simulink model "main"  (R2020a)
settings: Solver=FixedStepAuto  StartTime=0.0  StopTime=500  FixedStep=1e-3  RelTol=1e-3
values from neighbouring files (symbols this model uses):
  A = 2.5437    [configuracion.m]
  Cd = 0.31    [configuracion.m]
  d0 = 200    [configuracion.m]
  f = 0.02    [configuracion.m]
  F0 = m*g*sin(theta0)+f*m*g*cos(theta0)+(rho*Cd*A*(v0+w0)^2)/2    [configuracion.m]
  g = 9.81    [configuracion.m]
  K = 1/(rho*Cd*A*(v0+w0))    (= 0.0479562557583)    [configuracion.m]
  K_acc = place(Ac,Bc,p)    [configuracion.m]
  Kp = tau/(tau_bc*K)    (= 100)    [configuracion.m]
  m = 1500    [configuracion.m]
  rho = 1.202    [configuracion.m]
  tau = m/(rho*Cd*A*(v0+w0))    (= 71.9343836374)    [configuracion.m]
  Ti = tau    (= 71.9343836374)    [configuracion.m]
  v0 = 20    [configuracion.m]
libraries: simulink x10
settings Model: PacingRate=0.500000  Creator=FARUMO-SRM  LastModifiedBy=FARUMO-SRM

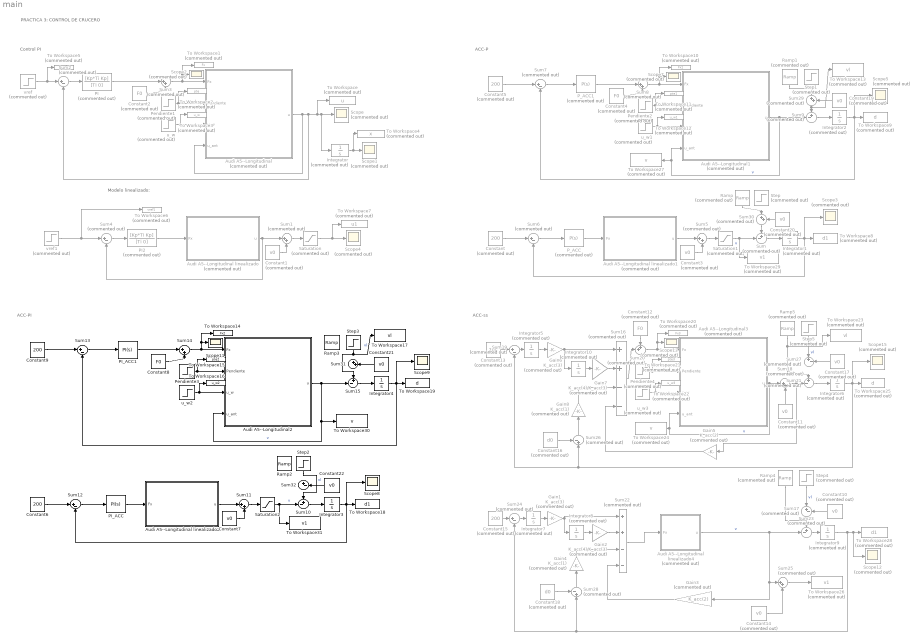
== system main ==
  note: ACC-P
  note: Control PI
  note: PRACTICA 3: CONTROL DE CRUCERO
  note: Modelo linealizado:
  note: ACC-PI
  note: ACC-ss
  Audi A5--Longitudinal : Subsystem  Commented=on
  Audi A5--Longitudinal linealizado : Subsystem  Commented=on
  Audi A5--Longitudinal linealizado1 : Subsystem  Commented=on
  Audi A5--Longitudinal linealizado2 : Subsystem
  Audi A5--Longitudinal linealizado4 : Subsystem  Commented=on
  Audi A5--Longitudinal1 : Subsystem  Commented=on
  Audi A5--Longitudinal2 : Subsystem
  Audi A5--Longitudinal3 : Subsystem  Commented=on
  Constant{,5,13,15} (4 alike) : Constant  Commented=on  Value=200
  Constant{1,3,10..11,14,17,19..20} (8 alike) : Constant  Commented=on  Value=v0
  Constant12 : Constant  Commented=on  Value=F0
  Constant16 : Constant  Commented=on  Value=d0
  Constant18 : Constant  Commented=on  Value=d0
  Constant2 : Constant  Commented=on  Value=F0
  Constant21 : Constant  Value=v0
  Constant22 : Constant  Value=v0
  Constant4 : Constant  Commented=on  Value=F0
  Constant6 : Constant  Value=200
  Constant7 : Constant  Value=v0
  Constant8 : Constant  Value=F0
  Constant9 : Constant  Value=200
  Gain1 : Gain  Commented=on  Gain=K_acc(3)
  Gain2 : Gain  Commented=on  Gain=K_acc(4)/K_acc(3)
  Gain3 : Gain  Commented=on  Gain=K_acc(2)
  Gain4 : Gain  Commented=on  Gain=K_acc(1)
  Gain5 : Gain  Commented=on  Gain=K_acc(2)
  Gain6 : Gain  Commented=on  Gain=K_acc(3)
  Gain7 : Gain  Commented=on  Gain=K_acc(4)/K_acc(3)
  Gain8 : Gain  Commented=on  Gain=K_acc(1)
  Integrator{,5,7..8,10} (5 alike) : Integrator  Commented=on
  Integrator{1..2,6,9} (4 alike) : Integrator  Commented=on  InitialCondition=200
  Integrator3 : Integrator  InitialCondition=200
  Integrator4 : Integrator  InitialCondition=200
  PI : TransferFcn  Commented=on  Numerator=[Kp*Ti Kp]  Denominator=[Ti 0]
  PI2 : TransferFcn  Commented=on  Numerator=[Kp*Ti Kp]  Denominator=[Ti 0]
  PI_ACC : simulink/Continuous/PID Controller  Controller=PI  Form=Parallel  TimeDomain=Continuous-time  UseExternalTs=off  SampleTime=-1  IntegratorMethod=Forward Euler  FilterMethod=Forward Euler  ControllerParametersSource=internal  P=-43.17834467421512  I=-0.01250307588771904  D=0  UseFilter=on  N=100  TunerSelectOption=Transfer Function Based (PID Tuner App)  InitialConditionSource=internal  InitialConditionForIntegrator=0  InitialConditionForFilter=0  DifferentiatorICPrevScaledInput=0  ExternalReset=none  TrackingMode=off  Kt=1  LimitOutput=off  UpperSaturationLimit=inf  LowerSaturationLimit=-inf  LinearizeAsGain=on  AntiWindupMode=none  Kb=1  POutMin=[]  POutMax=[]  IOutMin=[]  IOutMax=[]  DOutMin=[]  DOutMax=[]  NOutMin=[]  NOutMax=[]  SumOutMin=[]  SumOutMax=[]  SaturationOutMin=[]  SaturationOutMax=[]  PParamMin=[]  PParamMax=[]  IParamMin=[]  IParamMax=[]  DParamMin=[]  DParamMax=[]  NParamMin=[]  NParamMax=[]  KbParamMin=[]  KbParamMax=[]  KtParamMin=[]  KtParamMax=[]  KbOutMin=[]  KbOutMax=[]  KtOutMin=[]  KtOutMax=[]  IntegratorOutMin=[]  IntegratorOutMax=[]  FilterOutMin=[]  FilterOutMax=[]  SumI1OutMin=[]  SumI1OutMax=[]  SumI2OutMin=[]  SumI2OutMax=[]  SumI3OutMin=[]  SumI3OutMax=[]  SumI4OutMin=[]  SumI4OutMax=[]  SumDOutMin=[]  SumDOutMax=[]  DifferentiatorOutMin=[]  DifferentiatorOutMax=[]  FilterDiffOutCoefMin=[]  FilterDiffOutCoefMax=[]  ReciprocalOutMin=[]  ReciprocalOutMax=[]  SumDenOutMin=[]  SumDenOutMax=[]  SumNumOutMin=[]  SumNumOutMax=[]  DivideOutMin=[]  DivideOutMax=[]  UdiffTsProdOutMin=[]  UdiffTsProdOutMax=[]  NTsProdOutMin=[]  NTsProdOutMax=[]  UintegralTsProdOutMin=[]  UintegralTsProdOutMax=[]  UngainTsProdOutMin=[]  UngainTsProdOutMax=[]  IntegratorContinuousStateAttributes=''  IntegratorStateMustResolveToSignalObject=off  IntegratorRTWStateStorageClass=Auto  FilterContinuousStateAttributes=''  FilterStateMustResolveToSignalObject=off  FilterRTWStateStorageClass=Auto  ParallelPVariant=InternalParameters  IdealPVariant=Disabled  IVariant=InternalParameters  DVariant=Disabled  IntegratorVariant=Continuous  SatVariant=Disabled  AWVariant=Passthrough  PCopyVariant=Disabled  TRVariant=Disabled  FdbkBlocksVariant=Forward  IdealPFdbkVariant=Disabled  SatFdbkVariant=Disabled  DerivativeFilterVariant=Disabled  NVariant=Disabled  NCopyVariant=Disabled_SignalSpec  FilterICVariant=Disabled  IntegratorICVariant=InternalICs  ExternalResetVariant=Disabled  TRSumVariant=Passthrough  SumFdbkVariant=Disabled  SumVariant=Sum_PI  TsampFilterVariant=InternalTs  TsampNgainVariant=Passthrough  TsampIntegralVariant=Passthrough
  PI_ACC1 : simulink/Continuous/PID Controller  Controller=PI  Form=Parallel  TimeDomain=Continuous-time  UseExternalTs=off  SampleTime=-1  IntegratorMethod=Forward Euler  FilterMethod=Forward Euler  ControllerParametersSource=internal  P=-43.17834467421512  I=-0.01250307588771904  D=0  UseFilter=on  N=100  TunerSelectOption=Transfer Function Based (PID Tuner App)  InitialConditionSource=internal  InitialConditionForIntegrator=0  InitialConditionForFilter=0  DifferentiatorICPrevScaledInput=0  ExternalReset=none  TrackingMode=off  Kt=1  LimitOutput=off  UpperSaturationLimit=inf  LowerSaturationLimit=-inf  LinearizeAsGain=on  AntiWindupMode=none  Kb=1  POutMin=[]  POutMax=[]  IOutMin=[]  IOutMax=[]  DOutMin=[]  DOutMax=[]  NOutMin=[]  NOutMax=[]  SumOutMin=[]  SumOutMax=[]  SaturationOutMin=[]  SaturationOutMax=[]  PParamMin=[]  PParamMax=[]  IParamMin=[]  IParamMax=[]  DParamMin=[]  DParamMax=[]  NParamMin=[]  NParamMax=[]  KbParamMin=[]  KbParamMax=[]  KtParamMin=[]  KtParamMax=[]  KbOutMin=[]  KbOutMax=[]  KtOutMin=[]  KtOutMax=[]  IntegratorOutMin=[]  IntegratorOutMax=[]  FilterOutMin=[]  FilterOutMax=[]  SumI1OutMin=[]  SumI1OutMax=[]  SumI2OutMin=[]  SumI2OutMax=[]  SumI3OutMin=[]  SumI3OutMax=[]  SumI4OutMin=[]  SumI4OutMax=[]  SumDOutMin=[]  SumDOutMax=[]  DifferentiatorOutMin=[]  DifferentiatorOutMax=[]  FilterDiffOutCoefMin=[]  FilterDiffOutCoefMax=[]  ReciprocalOutMin=[]  ReciprocalOutMax=[]  SumDenOutMin=[]  SumDenOutMax=[]  SumNumOutMin=[]  SumNumOutMax=[]  DivideOutMin=[]  DivideOutMax=[]  UdiffTsProdOutMin=[]  UdiffTsProdOutMax=[]  NTsProdOutMin=[]  NTsProdOutMax=[]  UintegralTsProdOutMin=[]  UintegralTsProdOutMax=[]  UngainTsProdOutMin=[]  UngainTsProdOutMax=[]  IntegratorContinuousStateAttributes=''  IntegratorStateMustResolveToSignalObject=off  IntegratorRTWStateStorageClass=Auto  FilterContinuousStateAttributes=''  FilterStateMustResolveToSignalObject=off  FilterRTWStateStorageClass=Auto  ParallelPVariant=InternalParameters  IdealPVariant=Disabled  IVariant=InternalParameters  DVariant=Disabled  IntegratorVariant=Continuous  SatVariant=Disabled  AWVariant=Passthrough  PCopyVariant=Disabled  TRVariant=Disabled  FdbkBlocksVariant=Forward  IdealPFdbkVariant=Disabled  SatFdbkVariant=Disabled  DerivativeFilterVariant=Disabled  NVariant=Disabled  NCopyVariant=Disabled_SignalSpec  FilterICVariant=Disabled  IntegratorICVariant=InternalICs  ExternalResetVariant=Disabled  TRSumVariant=Passthrough  SumFdbkVariant=Disabled  SumVariant=Sum_PI  TsampFilterVariant=InternalTs  TsampNgainVariant=Passthrough  TsampIntegralVariant=Passthrough
  P_ACC : simulink/Continuous/PID Controller  Commented=on  Controller=P  Form=Parallel  TimeDomain=Continuous-time  UseExternalTs=off  SampleTime=-1  IntegratorMethod=Forward Euler  FilterMethod=Forward Euler  ControllerParametersSource=internal  P=-8.95543777959224  I=1  D=0  UseFilter=on  N=100  TunerSelectOption=Transfer Function Based (PID Tuner App)  InitialConditionSource=internal  InitialConditionForIntegrator=0  InitialConditionForFilter=0  DifferentiatorICPrevScaledInput=0  ExternalReset=none  TrackingMode=off  Kt=1  LimitOutput=off  UpperSaturationLimit=inf  LowerSaturationLimit=-inf  LinearizeAsGain=on  AntiWindupMode=none  Kb=1  POutMin=[]  POutMax=[]  IOutMin=[]  IOutMax=[]  DOutMin=[]  DOutMax=[]  NOutMin=[]  NOutMax=[]  SumOutMin=[]  SumOutMax=[]  SaturationOutMin=[]  SaturationOutMax=[]  PParamMin=[]  PParamMax=[]  IParamMin=[]  IParamMax=[]  DParamMin=[]  DParamMax=[]  NParamMin=[]  NParamMax=[]  KbParamMin=[]  KbParamMax=[]  KtParamMin=[]  KtParamMax=[]  KbOutMin=[]  KbOutMax=[]  KtOutMin=[]  KtOutMax=[]  IntegratorOutMin=[]  IntegratorOutMax=[]  FilterOutMin=[]  FilterOutMax=[]  SumI1OutMin=[]  SumI1OutMax=[]  SumI2OutMin=[]  SumI2OutMax=[]  SumI3OutMin=[]  SumI3OutMax=[]  SumI4OutMin=[]  SumI4OutMax=[]  SumDOutMin=[]  SumDOutMax=[]  DifferentiatorOutMin=[]  DifferentiatorOutMax=[]  FilterDiffOutCoefMin=[]  FilterDiffOutCoefMax=[]  ReciprocalOutMin=[]  ReciprocalOutMax=[]  SumDenOutMin=[]  SumDenOutMax=[]  SumNumOutMin=[]  SumNumOutMax=[]  DivideOutMin=[]  DivideOutMax=[]  UdiffTsProdOutMin=[]  UdiffTsProdOutMax=[]  NTsProdOutMin=[]  NTsProdOutMax=[]  UintegralTsProdOutMin=[]  UintegralTsProdOutMax=[]  UngainTsProdOutMin=[]  UngainTsProdOutMax=[]  IntegratorContinuousStateAttributes=''  IntegratorStateMustResolveToSignalObject=off  IntegratorRTWStateStorageClass=Auto  FilterContinuousStateAttributes=''  FilterStateMustResolveToSignalObject=off  FilterRTWStateStorageClass=Auto  ParallelPVariant=InternalParameters  IdealPVariant=Disabled  IVariant=Disabled  DVariant=Disabled  IntegratorVariant=Disabled  SatVariant=Disabled  AWVariant=Disabled  PCopyVariant=Disabled  TRVariant=Disabled  FdbkBlocksVariant=Forward  IdealPFdbkVariant=Disabled  SatFdbkVariant=Disabled  DerivativeFilterVariant=Disabled  NVariant=Disabled  NCopyVariant=Disabled_SignalSpec  FilterICVariant=Disabled  IntegratorICVariant=Disabled  ExternalResetVariant=Disabled  TRSumVariant=Passthrough  SumFdbkVariant=Disabled  SumVariant=Passthrough_P  TsampFilterVariant=InternalTs  TsampNgainVariant=Passthrough  TsampIntegralVariant=Disabled_SignalSpec
  P_ACC1 : simulink/Continuous/PID Controller  Commented=on  Controller=P  Form=Parallel  TimeDomain=Continuous-time  UseExternalTs=off  SampleTime=-1  IntegratorMethod=Forward Euler  FilterMethod=Forward Euler  ControllerParametersSource=internal  P=-8.95543777959224  I=1  D=0  UseFilter=on  N=100  TunerSelectOption=Transfer Function Based (PID Tuner App)  InitialConditionSource=internal  InitialConditionForIntegrator=0  InitialConditionForFilter=0  DifferentiatorICPrevScaledInput=0  ExternalReset=none  TrackingMode=off  Kt=1  LimitOutput=off  UpperSaturationLimit=inf  LowerSaturationLimit=-inf  LinearizeAsGain=on  AntiWindupMode=none  Kb=1  POutMin=[]  POutMax=[]  IOutMin=[]  IOutMax=[]  DOutMin=[]  DOutMax=[]  NOutMin=[]  NOutMax=[]  SumOutMin=[]  SumOutMax=[]  SaturationOutMin=[]  SaturationOutMax=[]  PParamMin=[]  PParamMax=[]  IParamMin=[]  IParamMax=[]  DParamMin=[]  DParamMax=[]  NParamMin=[]  NParamMax=[]  KbParamMin=[]  KbParamMax=[]  KtParamMin=[]  KtParamMax=[]  KbOutMin=[]  KbOutMax=[]  KtOutMin=[]  KtOutMax=[]  IntegratorOutMin=[]  IntegratorOutMax=[]  FilterOutMin=[]  FilterOutMax=[]  SumI1OutMin=[]  SumI1OutMax=[]  SumI2OutMin=[]  SumI2OutMax=[]  SumI3OutMin=[]  SumI3OutMax=[]  SumI4OutMin=[]  SumI4OutMax=[]  SumDOutMin=[]  SumDOutMax=[]  DifferentiatorOutMin=[]  DifferentiatorOutMax=[]  FilterDiffOutCoefMin=[]  FilterDiffOutCoefMax=[]  ReciprocalOutMin=[]  ReciprocalOutMax=[]  SumDenOutMin=[]  SumDenOutMax=[]  SumNumOutMin=[]  SumNumOutMax=[]  DivideOutMin=[]  DivideOutMax=[]  UdiffTsProdOutMin=[]  UdiffTsProdOutMax=[]  NTsProdOutMin=[]  NTsProdOutMax=[]  UintegralTsProdOutMin=[]  UintegralTsProdOutMax=[]  UngainTsProdOutMin=[]  UngainTsProdOutMax=[]  IntegratorContinuousStateAttributes=''  IntegratorStateMustResolveToSignalObject=off  IntegratorRTWStateStorageClass=Auto  FilterContinuousStateAttributes=''  FilterStateMustResolveToSignalObject=off  FilterRTWStateStorageClass=Auto  ParallelPVariant=InternalParameters  IdealPVariant=Disabled  IVariant=Disabled  DVariant=Disabled  IntegratorVariant=Disabled  SatVariant=Disabled  AWVariant=Disabled  PCopyVariant=Disabled  TRVariant=Disabled  FdbkBlocksVariant=Forward  IdealPFdbkVariant=Disabled  SatFdbkVariant=Disabled  DerivativeFilterVariant=Disabled  NVariant=Disabled  NCopyVariant=Disabled_SignalSpec  FilterICVariant=Disabled  IntegratorICVariant=Disabled  ExternalResetVariant=Disabled  TRSumVariant=Passthrough  SumFdbkVariant=Disabled  SumVariant=Passthrough_P  TsampFilterVariant=InternalTs  TsampNgainVariant=Passthrough  TsampIntegralVariant=Disabled_SignalSpec
  Pendiente1 : Step  Commented=on  Time=50  After=0  SampleTime=0
  Pendiente2 : Step  Commented=on  Time=50  After=0  SampleTime=0
  Pendiente3 : Step  Time=50  After=0  SampleTime=0
  Pendiente4 : Step  Commented=on  Time=50  After=0  SampleTime=0
  Ramp{,1,4..5} (4 alike) : simulink/Sources/Ramp  Commented=on  slope=1  start=100  InitialOutput=0
  Ramp2 : simulink/Sources/Ramp  slope=1  start=100  InitialOutput=0
  Ramp3 : simulink/Sources/Ramp  slope=1  start=100  InitialOutput=0
  Saturation : Saturate  Commented=on  UpperLimit=inf  LowerLimit=0
  Saturation1 : Saturate  Commented=on  UpperLimit=inf  LowerLimit=0
  Saturation2 : Saturate  UpperLimit=inf  LowerLimit=0
  Scope{,1..5,7,12..13,15} (10 alike) : Scope  Commented=on
  Scope11 : Scope
  Scope8 : Scope
  Scope9 : Scope
  Step{,1,4..5} (4 alike) : Step  Commented=on  Time=100  Before=20  After=22  SampleTime=0
  Step2 : Step  Time=100  Before=20  After=22  SampleTime=0
  Step3 : Step  Time=100  Before=20  After=22  SampleTime=0
  Sum{,9,21,23} (4 alike) : Sum  Commented=on  Inputs=+-|
  Sum{1,3,5,8,25,29..30} (7 alike) : Sum  Commented=on  Inputs=|++
  Sum10 : Sum  Inputs=+-|
  Sum11 : Sum  Inputs=|++
  Sum12 : Sum  Inputs=|+-
  Sum13 : Sum  Inputs=|+-
  Sum14 : Sum  Inputs=|++
  Sum15 : Sum  Inputs=+-|
  Sum16 : Sum  Commented=on  Inputs=++--
  Sum{2,4,6..7,17..19,24,27} (9 alike) : Sum  Commented=on  Inputs=|+-
  Sum20 : Sum  Commented=on  Inputs=++|
  Sum22 : Sum  Commented=on  Inputs=++--
  Sum26 : Sum  Commented=on  Inputs=-+|
  Sum28 : Sum  Commented=on  Inputs=-+|
  Sum31 : Sum  Inputs=|++
  Sum32 : Sum  Inputs=|+-
  To Workspace : ToWorkspace  Commented=on  VariableName=u  SaveFormat=Timeseries  SampleTime=-1
  To Workspace1 : ToWorkspace  Commented=on  VariableName=Fx  SaveFormat=Timeseries  SampleTime=-1
  To Workspace10 : ToWorkspace  Commented=on  VariableName=Fx1  SaveFormat=Timeseries  SampleTime=-1
  To Workspace11 : ToWorkspace  Commented=on  VariableName=pte1  SaveFormat=Timeseries  SampleTime=-1
  To Workspace12 : ToWorkspace  Commented=on  VariableName=u_w1  SaveFormat=Timeseries  SampleTime=-1
  To Workspace13 : ToWorkspace  Commented=on  VariableName=vl  SaveFormat=Timeseries  SampleTime=-1
  To Workspace14 : ToWorkspace  VariableName=Fx2  SaveFormat=Timeseries  SampleTime=-1
  To Workspace15 : ToWorkspace  VariableName=pte2  SaveFormat=Timeseries  SampleTime=-1
  To Workspace16 : ToWorkspace  VariableName=u_w2  SaveFormat=Timeseries  SampleTime=-1
  To Workspace17 : ToWorkspace  VariableName=vl  SaveFormat=Timeseries  SampleTime=-1
  To Workspace18 : ToWorkspace  VariableName=d1  SaveFormat=Timeseries  SampleTime=-1
  To Workspace19 : ToWorkspace  VariableName=d  SaveFormat=Timeseries  SampleTime=-1
  To Workspace2 : ToWorkspace  Commented=on  VariableName=pte  SaveFormat=Timeseries  SampleTime=-1
  To Workspace20 : ToWorkspace  Commented=on  VariableName=Fx3  SaveFormat=Timeseries  SampleTime=-1
  To Workspace21 : ToWorkspace  Commented=on  VariableName=pte3  SaveFormat=Timeseries  SampleTime=-1
  To Workspace22 : ToWorkspace  Commented=on  VariableName=u_w3  SaveFormat=Timeseries  SampleTime=-1
  To Workspace23 : ToWorkspace  Commented=on  VariableName=vl  SaveFormat=Timeseries  SampleTime=-1
  To Workspace24 : ToWorkspace  Commented=on  VariableName=v  SaveFormat=Timeseries  SampleTime=-1
  To Workspace25 : ToWorkspace  Commented=on  VariableName=d  SaveFormat=Timeseries  SampleTime=-1
  To Workspace26 : ToWorkspace  Commented=on  VariableName=v1  SaveFormat=Timeseries  SampleTime=-1
  To Workspace27 : ToWorkspace  Commented=on  VariableName=v  SaveFormat=Timeseries  SampleTime=-1
  To Workspace28 : ToWorkspace  Commented=on  VariableName=d1  SaveFormat=Timeseries  SampleTime=-1
  To Workspace29 : ToWorkspace  Commented=on  VariableName=v1  SaveFormat=Timeseries  SampleTime=-1
  To Workspace3 : ToWorkspace  Commented=on  VariableName=u_w  SaveFormat=Timeseries  SampleTime=-1
  To Workspace30 : ToWorkspace  VariableName=v  SaveFormat=Timeseries  SampleTime=-1
  To Workspace31 : ToWorkspace  VariableName=v1  SaveFormat=Timeseries  SampleTime=-1
  To Workspace4 : ToWorkspace  Commented=on  VariableName=x  SaveFormat=Timeseries  SampleTime=-1
  To Workspace5 : ToWorkspace  Commented=on  VariableName=vref  SaveFormat=Timeseries  SampleTime=-1
  To Workspace6 : ToWorkspace  Commented=on  VariableName=vref1  SaveFormat=Timeseries  SampleTime=-1
  To Workspace7 : ToWorkspace  Commented=on  VariableName=u1  SaveFormat=Timeseries  SampleTime=-1
  To Workspace8 : ToWorkspace  Commented=on  VariableName=d1  SaveFormat=Timeseries  SampleTime=-1
  To Workspace9 : ToWorkspace  Commented=on  VariableName=d  SaveFormat=Timeseries  SampleTime=-1
  u_w : Step  Commented=on  Time=50  Before=2  After=2  SampleTime=0
  u_w1 : Step  Commented=on  Time=50  Before=2  After=2  SampleTime=0
  u_w2 : Step  Time=50  Before=2  After=2  SampleTime=0
  u_w3 : Step  Commented=on  Time=50  Before=2  After=2  SampleTime=0
  vref : Step  Commented=on  Time=50  Before=20  After=30  SampleTime=0
  vref1 : Step  Commented=on  Time=50  After=10  SampleTime=0
  wires:
  u_w/1 -> Audi A5--Longitudinal/3(u_w), To Workspace3/1
  Pendiente1/1 -> To Workspace2/1, Audi A5--Longitudinal/2(Pendiente)
  Integrator/1 -> To Workspace4/1, Scope1/1
  Sum2/1 -> PI/1
  Sum1/1 -> Saturation/1
  Constant1/1 -> Sum1/2
  Saturation/1 -> To Workspace7/1, Scope4/1
  vref/1 -> To Workspace5/1, Sum2/1
  Audi A5--Longitudinal/1(u) -> Sum2/2, To Workspace/1, Integrator/1, Scope/1, Audi A5--Longitudinal/4(u_ant)
  PI/1 -> Sum3/1
  Sum3/1 -> To Workspace1/1, Scope2/1, Audi A5--Longitudinal/1(Fx)
  Constant2/1 -> Sum3/2
  Audi A5--Longitudinal linealizado/1(u) -> Sum1/1, Sum4/2
  vref1/1 -> Sum4/1, To Workspace6/1
  Sum4/1 -> PI2/1
  PI2/1 -> Audi A5--Longitudinal linealizado/1(Fx)
  Constant3/1 -> Sum5/2
  Sum5/1 -> Saturation1/1
  Saturation1/1 -> To Workspace29/1, Sum/2  "v"
  Audi A5--Longitudinal linealizado1/1(u) -> Sum5/1
  Sum/1 -> Integrator1/1
  Integrator1/1 -> Scope3/1, Sum6/2, To Workspace8/1
  P_ACC/1 -> Audi A5--Longitudinal linealizado1/1(Fx)
  Sum6/1 -> P_ACC/1
  Constant/1 -> Sum6/1
  Sum8/1 -> To Workspace10/1, Scope7/1, Audi A5--Longitudinal1/1(Fx)
  Constant4/1 -> Sum8/2
  P_ACC1/1 -> Sum8/1
  Constant5/1 -> Sum7/1
  Sum7/1 -> P_ACC1/1
  Pendiente2/1 -> To Workspace11/1, Audi A5--Longitudinal1/2(Pendiente)
  u_w1/1 -> Audi A5--Longitudinal1/3(u_w), To Workspace12/1
  Integrator2/1 -> Sum7/2, Scope5/1, To Workspace9/1
  Audi A5--Longitudinal1/1(u) -> Sum9/2, To Workspace27/1, Audi A5--Longitudinal1/4(u_ant)  "v"
  Sum9/1 -> Integrator2/1
  Sum12/1 -> PI_ACC/1
  Sum13/1 -> PI_ACC1/1
  Sum15/1 -> Integrator4/1
  Sum10/1 -> Integrator3/1
  Audi A5--Longitudinal2/1(u) -> Sum15/2, To Workspace30/1, Audi A5--Longitudinal2/4(u_ant)  "v"
  Audi A5--Longitudinal linealizado2/1(u) -> Sum11/1
  Constant9/1 -> Sum13/1
  u_w2/1 -> Audi A5--Longitudinal2/3(u_w), To Workspace16/1
  PI_ACC/1 -> Audi A5--Longitudinal linealizado2/1(Fx)
  Pendiente3/1 -> To Workspace15/1, Audi A5--Longitudinal2/2(Pendiente)
  Integrator4/1 -> Sum13/2, Scope9/1, To Workspace19/1
  Constant8/1 -> Sum14/2
  Sum14/1 -> To Workspace14/1, Scope11/1, Audi A5--Longitudinal2/1(Fx)
  Integrator3/1 -> Scope8/1, Sum12/2, To Workspace18/1
  Constant6/1 -> Sum12/1
  Sum11/1 -> Saturation2/1
  PI_ACC1/1 -> Sum14/1
  Constant7/1 -> Sum11/2
  Saturation2/1 -> To Workspace31/1, Sum10/2  "v"
  Audi A5--Longitudinal3/1(u) -> Sum18/1, Audi A5--Longitudinal3/4(u_ant), To Workspace24/1  "v"
  Sum20/1 -> To Workspace20/1, Scope13/1, Audi A5--Longitudinal3/1(Fx)
  Pendiente4/1 -> To Workspace21/1, Audi A5--Longitudinal3/2(Pendiente)
  Constant13/1 -> Sum19/1
  u_w3/1 -> Audi A5--Longitudinal3/3(u_w), To Workspace22/1
  Sum21/1 -> Integrator6/1
  Sum19/1 -> Integrator5/1
  Sum24/1 -> Integrator7/1
  Integrator9/1 -> Sum28/2, Sum24/2, Scope12/1, To Workspace28/1
  Integrator7/1 -> Gain1/1
  Constant15/1 -> Sum24/1
  Gain3/1 -> Sum22/4
  Sum23/1 -> Integrator9/1
  Gain4/1 -> Sum22/3
  Sum22/1 -> Audi A5--Longitudinal linealizado4/1(Fx)
  Integrator8/1 -> Gain2/1
  Audi A5--Longitudinal linealizado4/1(u) -> Sum25/1, Gain3/1, Sum23/2  "v"
  Integrator6/1 -> Sum26/2, Sum19/2, Scope15/1, To Workspace25/1
  Gain7/1 -> Sum16/2
  Integrator5/1 -> Gain6/1
  Integrator10/1 -> Gain7/1
  Gain5/1 -> Sum16/4
  Gain8/1 -> Sum16/3
  Gain1/1 -> Sum22/1, Integrator8/1
  Gain6/1 -> Sum16/1, Integrator10/1
  Sum16/1 -> Sum20/2
  Gain2/1 -> Sum22/2
  Sum18/1 -> Gain5/1, Sum21/2
  Constant11/1 -> Sum18/2
  Sum26/1 -> Gain8/1
  Constant12/1 -> Sum20/1
  Constant16/1 -> Sum26/1
  Constant17/1 -> Sum27/2
  Constant18/1 -> Sum28/1
  Sum28/1 -> Gain4/1
  Constant10/1 -> Sum17/2
  Step4/1 -> Sum17/1  "vl"
  Constant14/1 -> Sum25/2
  Sum25/1 -> To Workspace26/1
  Step5/1 -> Sum27/1  "vl"
  Constant19/1 -> Sum29/2
  Ramp5/1 -> Sum21/1, To Workspace23/1
  Ramp4/1 -> Sum23/1
  Ramp1/1 -> Sum29/1
  Sum29/1 -> To Workspace13/1, Sum9/1
  Ramp/1 -> Sum30/1
  Sum30/1 -> Sum/1
  Constant20/1 -> Sum30/2
  Constant21/1 -> Sum31/2
  Constant22/1 -> Sum32/2
  Step3/1 -> Sum15/1, To Workspace17/1  "vl"
  Step2/1 -> Sum10/1  "vl"

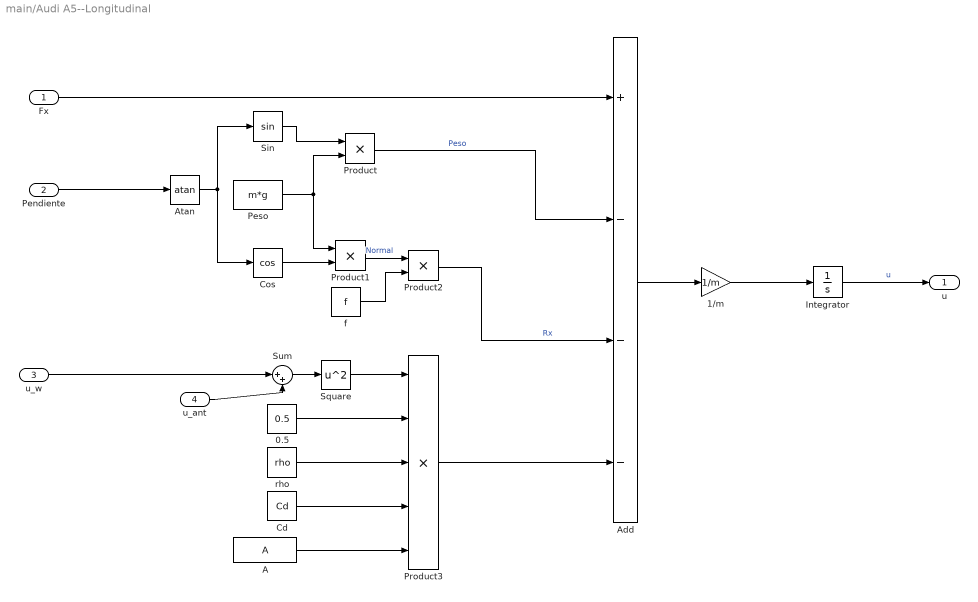
== system main/Audi A5--Longitudinal ==
  Fx : Inport
  Pendiente : Inport  Port=2
  u_w : Inport  Port=3
  u_ant : Inport  Port=4
  0.5 : Constant  Value=0.5
  1/m : Gain  Gain=1/m
  A : Constant  Value=A
  Add : Sum  Inputs=+---
  Atan : Trigonometry  Operator=atan
  Cd : Constant  Value=Cd
  Cos : Trigonometry  Operator=cos
  Integrator : Integrator  InitialCondition=v0  LimitOutput=on  LowerSaturationLimit=0
  Peso : Constant  Value=m*g
  Product : Product
  Product1 : Product
  Product2 : Product
  Product3 : Product  Inputs=5
  Sin : Trigonometry
  Square : Math  Operator=square  SaturateOnIntegerOverflow=on
  Sum : Sum  Inputs=|++
  f : Constant  Value=f
  rho : Constant  Value=rho
  u : Outport
  wires:
  Square/1 -> Product3/1
  Peso/1 -> Product1/1, Product/2
  Sin/1 -> Product/1
  Product2/1 -> Add/3  "Rx"
  A/1 -> Product3/5
  Product/1 -> Add/2  "Peso"
  Cd/1 -> Product3/4
  rho/1 -> Product3/3
  Product1/1 -> Product2/1  "Normal"
  Cos/1 -> Product1/2
  f/1 -> Product2/2
  0.5/1 -> Product3/2
  Sum/1 -> Square/1
  Product3/1 -> Add/4
  Fx/1 -> Add/1
  u_w/1 -> Sum/1
  u_ant/1 -> Sum/2
  Add/1 -> 1/m/1
  1/m/1 -> Integrator/1
  Integrator/1 -> u/1  "u"
  Pendiente/1 -> Atan/1
  Atan/1 -> Cos/1, Sin/1

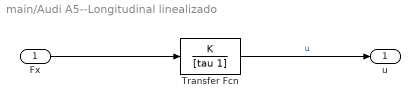
== system main/Audi A5--Longitudinal linealizado ==
  Fx : Inport
  Transfer Fcn : TransferFcn  Numerator=K  Denominator=[tau 1]
  u : Outport
  wires:
  Fx/1 -> Transfer Fcn/1
  Transfer Fcn/1 -> u/1  "u"

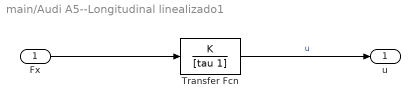
== system main/Audi A5--Longitudinal linealizado1 ==
  Fx : Inport
  Transfer Fcn : TransferFcn  Numerator=K  Denominator=[tau 1]
  u : Outport
  wires:
  Fx/1 -> Transfer Fcn/1
  Transfer Fcn/1 -> u/1  "u"

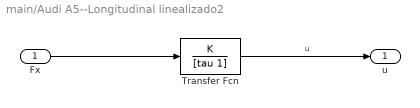
== system main/Audi A5--Longitudinal linealizado2 ==
  Fx : Inport
  Transfer Fcn : TransferFcn  Numerator=K  Denominator=[tau 1]
  u : Outport
  wires:
  Fx/1 -> Transfer Fcn/1
  Transfer Fcn/1 -> u/1  "u"

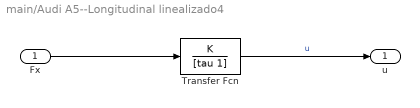
== system main/Audi A5--Longitudinal linealizado4 ==
  Fx : Inport
  Transfer Fcn : TransferFcn  Numerator=K  Denominator=[tau 1]
  u : Outport
  wires:
  Fx/1 -> Transfer Fcn/1
  Transfer Fcn/1 -> u/1  "u"

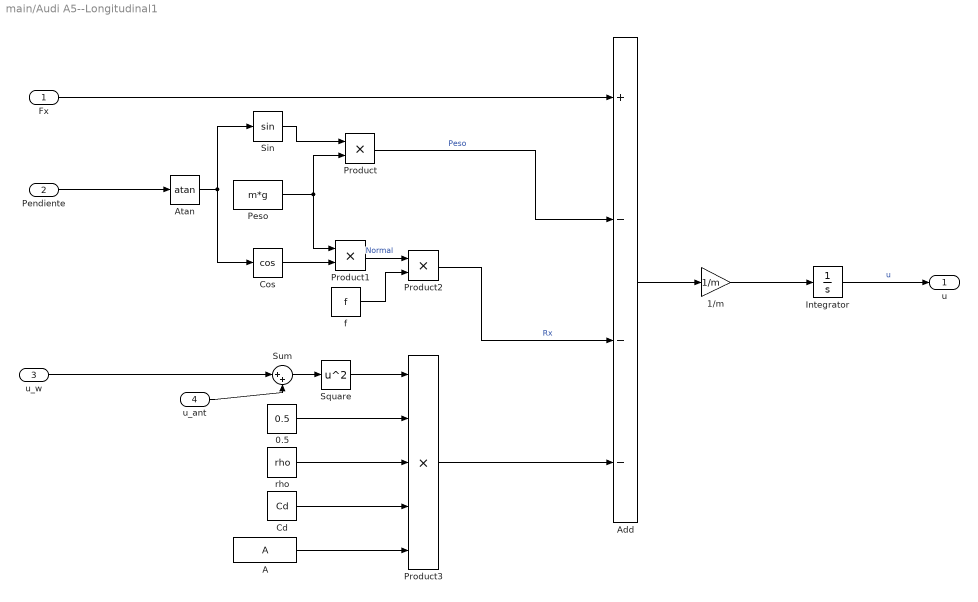
== system main/Audi A5--Longitudinal1 ==
  Fx : Inport
  Pendiente : Inport  Port=2
  u_w : Inport  Port=3
  u_ant : Inport  Port=4
  0.5 : Constant  Value=0.5
  1/m : Gain  Gain=1/m
  A : Constant  Value=A
  Add : Sum  Inputs=+---
  Atan : Trigonometry  Operator=atan
  Cd : Constant  Value=Cd
  Cos : Trigonometry  Operator=cos
  Integrator : Integrator  InitialCondition=v0  LimitOutput=on  LowerSaturationLimit=0
  Peso : Constant  Value=m*g
  Product : Product
  Product1 : Product
  Product2 : Product
  Product3 : Product  Inputs=5
  Sin : Trigonometry
  Square : Math  Operator=square  SaturateOnIntegerOverflow=on
  Sum : Sum  Inputs=|++
  f : Constant  Value=f
  rho : Constant  Value=rho
  u : Outport
  wires:
  Square/1 -> Product3/1
  Peso/1 -> Product1/1, Product/2
  Sin/1 -> Product/1
  Product2/1 -> Add/3  "Rx"
  A/1 -> Product3/5
  Product/1 -> Add/2  "Peso"
  Cd/1 -> Product3/4
  rho/1 -> Product3/3
  Product1/1 -> Product2/1  "Normal"
  Cos/1 -> Product1/2
  f/1 -> Product2/2
  0.5/1 -> Product3/2
  Sum/1 -> Square/1
  Product3/1 -> Add/4
  Fx/1 -> Add/1
  u_w/1 -> Sum/1
  u_ant/1 -> Sum/2
  Add/1 -> 1/m/1
  1/m/1 -> Integrator/1
  Integrator/1 -> u/1  "u"
  Pendiente/1 -> Atan/1
  Atan/1 -> Cos/1, Sin/1

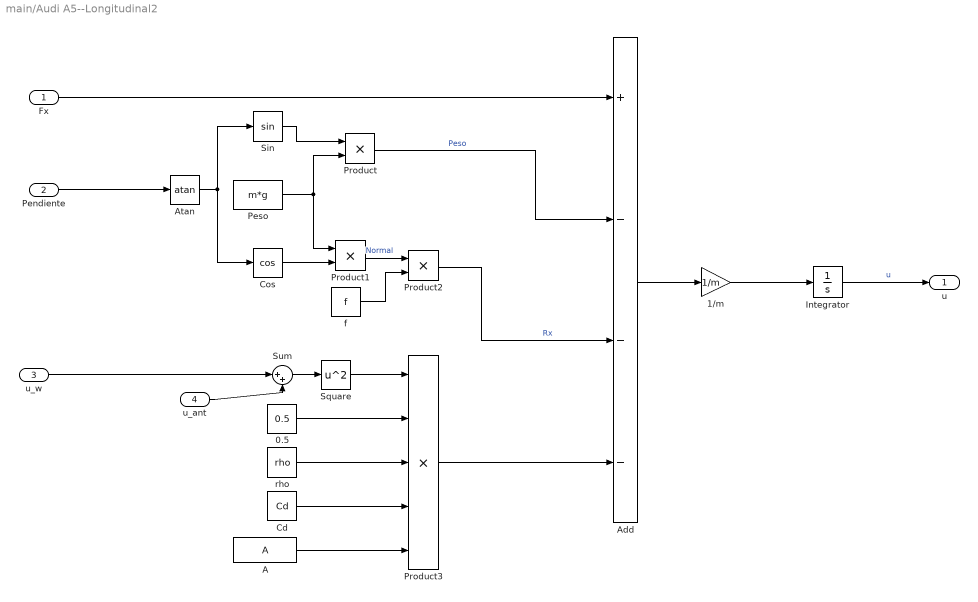
== system main/Audi A5--Longitudinal2 ==
  Fx : Inport
  Pendiente : Inport  Port=2
  u_w : Inport  Port=3
  u_ant : Inport  Port=4
  0.5 : Constant  Value=0.5
  1/m : Gain  Gain=1/m
  A : Constant  Value=A
  Add : Sum  Inputs=+---
  Atan : Trigonometry  Operator=atan
  Cd : Constant  Value=Cd
  Cos : Trigonometry  Operator=cos
  Integrator : Integrator  InitialCondition=v0  LimitOutput=on  LowerSaturationLimit=0
  Peso : Constant  Value=m*g
  Product : Product
  Product1 : Product
  Product2 : Product
  Product3 : Product  Inputs=5
  Sin : Trigonometry
  Square : Math  Operator=square  SaturateOnIntegerOverflow=on
  Sum : Sum  Inputs=|++
  f : Constant  Value=f
  rho : Constant  Value=rho
  u : Outport
  wires:
  Square/1 -> Product3/1
  Peso/1 -> Product1/1, Product/2
  Sin/1 -> Product/1
  Product2/1 -> Add/3  "Rx"
  A/1 -> Product3/5
  Product/1 -> Add/2  "Peso"
  Cd/1 -> Product3/4
  rho/1 -> Product3/3
  Product1/1 -> Product2/1  "Normal"
  Cos/1 -> Product1/2
  f/1 -> Product2/2
  0.5/1 -> Product3/2
  Sum/1 -> Square/1
  Product3/1 -> Add/4
  Fx/1 -> Add/1
  u_w/1 -> Sum/1
  u_ant/1 -> Sum/2
  Add/1 -> 1/m/1
  1/m/1 -> Integrator/1
  Integrator/1 -> u/1  "u"
  Pendiente/1 -> Atan/1
  Atan/1 -> Cos/1, Sin/1

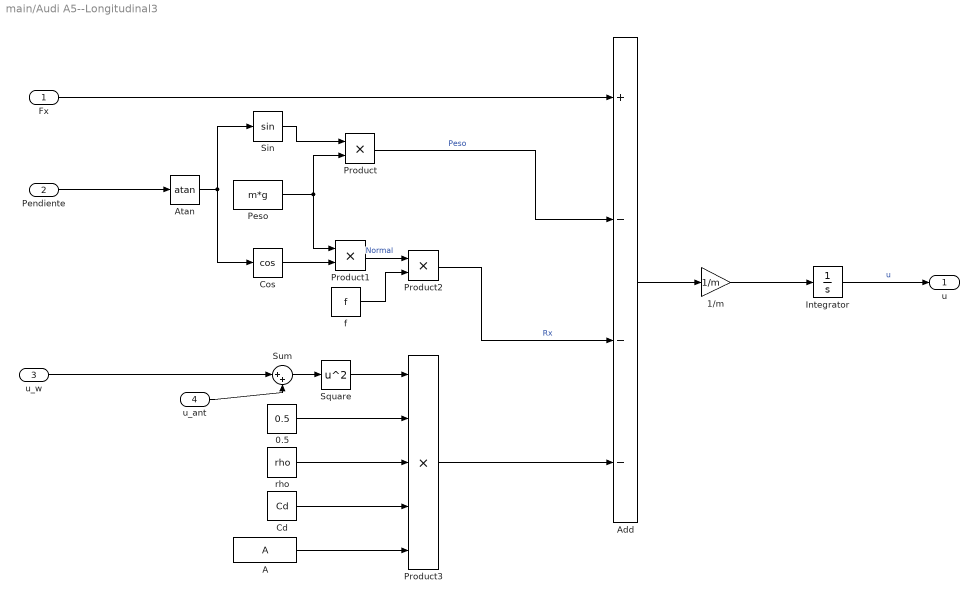
== system main/Audi A5--Longitudinal3 ==
  Fx : Inport
  Pendiente : Inport  Port=2
  u_w : Inport  Port=3
  u_ant : Inport  Port=4
  0.5 : Constant  Value=0.5
  1/m : Gain  Gain=1/m
  A : Constant  Value=A
  Add : Sum  Inputs=+---
  Atan : Trigonometry  Operator=atan
  Cd : Constant  Value=Cd
  Cos : Trigonometry  Operator=cos
  Integrator : Integrator  InitialCondition=v0  LimitOutput=on  LowerSaturationLimit=0
  Peso : Constant  Value=m*g
  Product : Product
  Product1 : Product
  Product2 : Product
  Product3 : Product  Inputs=5
  Sin : Trigonometry
  Square : Math  Operator=square  SaturateOnIntegerOverflow=on
  Sum : Sum  Inputs=|++
  f : Constant  Value=f
  rho : Constant  Value=rho
  u : Outport
  wires:
  Square/1 -> Product3/1
  Peso/1 -> Product1/1, Product/2
  Sin/1 -> Product/1
  Product2/1 -> Add/3  "Rx"
  A/1 -> Product3/5
  Product/1 -> Add/2  "Peso"
  Cd/1 -> Product3/4
  rho/1 -> Product3/3
  Product1/1 -> Product2/1  "Normal"
  Cos/1 -> Product1/2
  f/1 -> Product2/2
  0.5/1 -> Product3/2
  Sum/1 -> Square/1
  Product3/1 -> Add/4
  Fx/1 -> Add/1
  u_w/1 -> Sum/1
  u_ant/1 -> Sum/2
  Add/1 -> 1/m/1
  1/m/1 -> Integrator/1
  Integrator/1 -> u/1  "u"
  Pendiente/1 -> Atan/1
  Atan/1 -> Cos/1, Sin/1
